simulink model "LaserLight_Demo2"  (R2017b)
settings: Solver=VariableStepAuto  StartTime=0.0  StopTime=1  RelTol=1e-3
values from neighbouring files (symbols this model uses):
  BackEMF0 = 0.09331    [System.m]
  BackEMF1 = 0.001545    [System.m]
  D = 10    [CONSTANTS.m]
  Elec0d = [.00105 2.25]    [System.m]
  Elec0n = [1]    [System.m]
  Elec1d = [1]    [0Controller.m]    (also in System.m = [.00105 2.25])
  Elec1n = [1]    [0Controller.m]    (also in System.m)
  Mech0d = [1]    [0Controller.m]    (also in System.m = [0.0000002059 0.0000009585])
  Mech0n = [1]    [0Controller.m]    (also in System.m)
  Mech1d = [1]    [0Controller.m]    (also in System.m = [0.0000025152 0.00001854])
  Mech1n = [1]    [0Controller.m]    (also in System.m)
  TConst0 = 0.001574542    [System.m]
  TConst1 = 0.0193    [System.m]
libraries: simulink x6
settings Model: Creator=Jimmy  LastModifiedBy=jmvsu
settings CodeAppCC: StateflowObjectComments=on

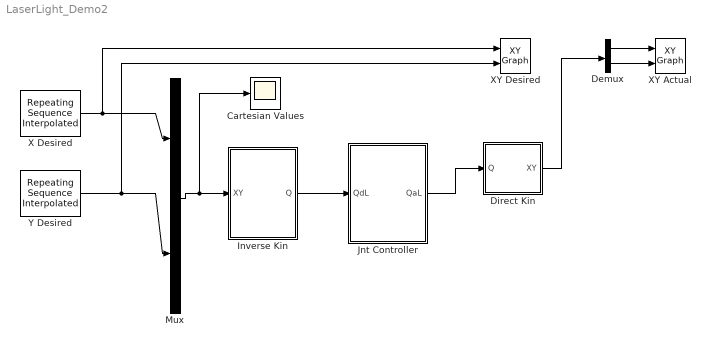
== system LaserLight_Demo2 ==
  Cartesian Values : Scope
  Demux : Demux  Outputs=2
  Direct Kin : Subsystem
  Inverse Kin : Subsystem
  Jnt Controller : Subsystem
  Mux : Mux  Inputs=2
  X Desired : simulink/Sources/Repeating Sequence Interpolated  OutValues=[100 100 -100 -100 100]  TimeValues=[0 0.25 0.5 0.75 1]  LookUpMeth=Interpolation-Use End Values  tsamp=0.01  OutMin=[]  OutMax=[]  OutDataTypeStr=double  OutputDataTypeScalingMode=double  OutDataType=fixdt(0,8)  OutScaling=2^-10
  XY Actual : simulink/Sinks/XY Graph  xmin=-125  xmax=125  ymin=-125  ymax=125  st=-1
  XY Desired : simulink/Sinks/XY Graph  xmin=-110  xmax=110  ymin=-110  ymax=110  st=-1
  Y Desired : simulink/Sources/Repeating Sequence Interpolated  OutValues=[-100 100 100 -100 -100]  TimeValues=[0 0.25 0.5 0.75 1]  LookUpMeth=Interpolation-Use End Values  tsamp=0.01  OutMin=[]  OutMax=[]  OutDataTypeStr=double  OutputDataTypeScalingMode=double  OutDataType=fixdt(0,8)  OutScaling=2^-10
  wires:
  Y Desired/1 -> XY Desired/2, Mux/2
  Demux/2 -> XY Actual/2
  Inverse Kin/1("Q ") -> Jnt Controller/1(QdL)
  Direct Kin/1(XY) -> Demux/1
  Jnt Controller/1(QaL) -> Direct Kin/1(Q)
  Demux/1 -> XY Actual/1
  Mux/1 -> Cartesian Values/1, Inverse Kin/1(XY)
  X Desired/1 -> Mux/1, XY Desired/1

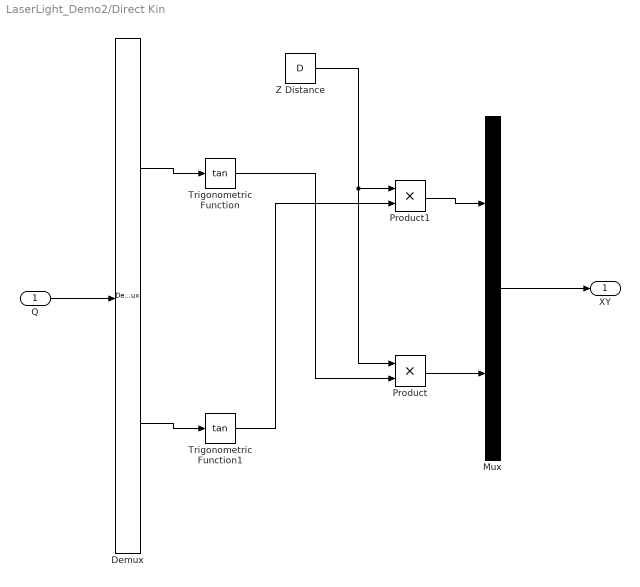
== system LaserLight_Demo2/Direct Kin ==
  Q : Inport
  Demux : Demux  Outputs=2
  Mux : Mux  Inputs=2
  Product : Product
  Product1 : Product
  Trigonometric Function : Trigonometry  Operator=tan
  Trigonometric Function1 : Trigonometry  Operator=tan
  Z Distance : Constant  Value=D
  XY : Outport
  wires:
  Q/1 -> Demux/1
  Mux/1 -> XY/1
  Demux/1 -> Trigonometric Function/1
  Demux/2 -> Trigonometric Function1/1
  Trigonometric Function/1 -> Product/2
  Z Distance/1 -> Product1/1, Product/1
  Trigonometric Function1/1 -> Product1/2
  Product1/1 -> Mux/1
  Product/1 -> Mux/2

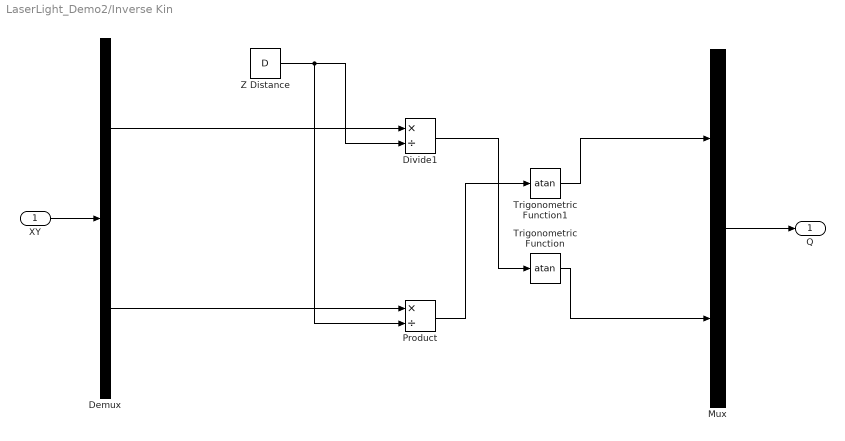
== system LaserLight_Demo2/Inverse Kin ==
  XY : Inport
  Demux : Demux  Outputs=2
  Divide1 : Product  Inputs=*/
  Mux : Mux  Inputs=2
  Product : Product  Inputs=*/
  Trigonometric Function : Trigonometry  Operator=atan
  Trigonometric Function1 : Trigonometry  Operator=atan
  "Z Distance " : Constant  Value=D
  "Q " : Outport
  wires:
  XY/1 -> Demux/1
  Mux/1 -> "Q "/1
  Demux/1 -> Divide1/1
  Trigonometric Function/1 -> Mux/2
  Divide1/1 -> Trigonometric Function/1
  "Z Distance "/1 -> Product/2, Divide1/2
  Demux/2 -> Product/1
  Trigonometric Function1/1 -> Mux/1
  Product/1 -> Trigonometric Function1/1

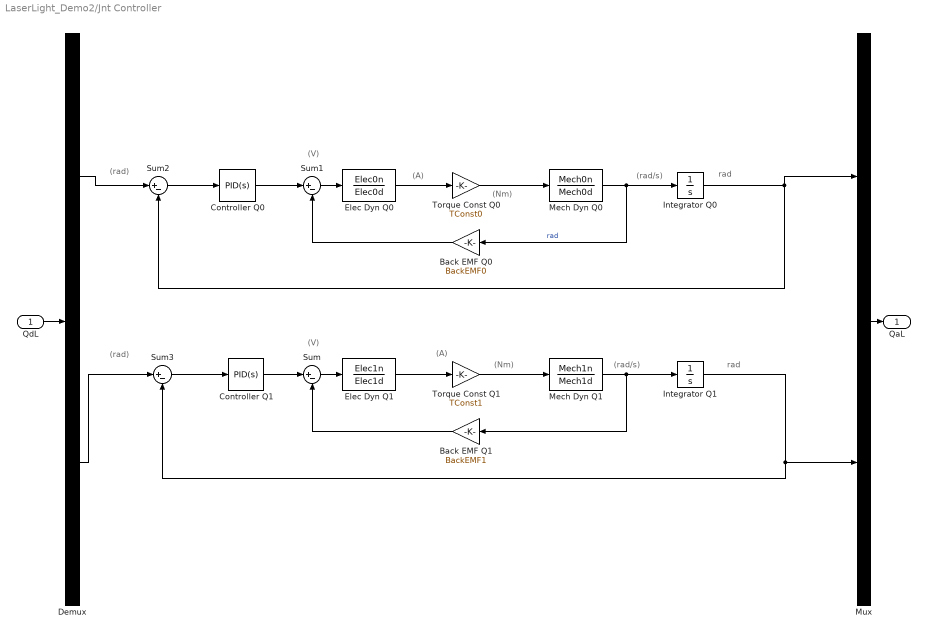
== system LaserLight_Demo2/Jnt Controller ==
  note: rad
  note: (rad/s)
  note: (V)
  note: (rad)
  note: (rad/s)
  note: (A)
  note: (Nm)
  note: (V)
  note: (A)
  note: (rad)
  note: (Nm)
  note: rad
  QdL : Inport
  Back EMF Q0 : Gain  Gain=BackEMF0
  Back EMF Q1 : Gain  Gain=BackEMF1
  Controller Q0 : simulink/Continuous/PID Controller  Controller=PID  TimeDomain=Continuous-time  SampleTime=-1  IntegratorMethod=Forward Euler  FilterMethod=Forward Euler  Form=Parallel  UseFilter=on  ControllerParametersSource=internal  P=1656.89310758008  I=104989.490543032  D=3.83138370012863  N=7457.36011167874  InitialConditionSource=internal  InitialConditionForIntegrator=0  InitialConditionForFilter=0  ExternalReset=none  LimitOutput=off  UpperSaturationLimit=inf  LowerSaturationLimit=-inf  LinearizeAsGain=on  AntiWindupMode=none  Kb=1  TrackingMode=off  Kt=1  PParamMin=[]  PParamMax=[]  IParamMin=[]  IParamMax=[]  DParamMin=[]  DParamMax=[]  NParamMin=[]  NParamMax=[]  KbParamMin=[]  KbParamMax=[]  KtParamMin=[]  KtParamMax=[]  POutMin=[]  POutMax=[]  IOutMin=[]  IOutMax=[]  DOutMin=[]  DOutMax=[]  NOutMin=[]  NOutMax=[]  KbOutMin=[]  KbOutMax=[]  KtOutMin=[]  KtOutMax=[]  IntegratorOutMin=[]  IntegratorOutMax=[]  FilterOutMin=[]  FilterOutMax=[]  SumOutMin=[]  SumOutMax=[]  SumI1OutMin=[]  SumI1OutMax=[]  SumI2OutMin=[]  SumI2OutMax=[]  SumI3OutMin=[]  SumI3OutMax=[]  SumDOutMin=[]  SumDOutMax=[]  SaturationOutMin=[]  SaturationOutMax=[]  IntegratorContinuousStateAttributes=''  IntegratorStateMustResolveToSignalObject=off  IntegratorRTWStateStorageClass=Auto  FilterContinuousStateAttributes=''  FilterStateMustResolveToSignalObject=off  FilterRTWStateStorageClass=Auto  DifferentiatorICPrevScaledInput=0  DifferentiatorOutMin=[]  DifferentiatorOutMax=[]  InitialConditionSetting=State (most efficient)  FilterDiffOutCoefMin=[]  FilterDiffOutCoefMax=[]  SumDenOutMin=[]  SumDenOutMax=[]  SumNumOutMin=[]  SumNumOutMax=[]  ReciprocalOutMin=[]  ReciprocalOutMax=[]  DivideOutMin=[]  DivideOutMax=[]  TunerSelectOption=Transfer Function Based (PID Tuner App)
  Controller Q1 : simulink/Continuous/PID Controller  Controller=PID  TimeDomain=Continuous-time  SampleTime=-1  IntegratorMethod=Forward Euler  FilterMethod=Forward Euler  Form=Parallel  UseFilter=on  ControllerParametersSource=internal  P=19.445961470142  I=200.878604706117  D=0.242603406733837  N=930.997703714061  InitialConditionSource=internal  InitialConditionForIntegrator=0  InitialConditionForFilter=0  ExternalReset=none  LimitOutput=off  UpperSaturationLimit=inf  LowerSaturationLimit=-inf  LinearizeAsGain=on  AntiWindupMode=none  Kb=1  TrackingMode=off  Kt=1  PParamMin=[]  PParamMax=[]  IParamMin=[]  IParamMax=[]  DParamMin=[]  DParamMax=[]  NParamMin=[]  NParamMax=[]  KbParamMin=[]  KbParamMax=[]  KtParamMin=[]  KtParamMax=[]  POutMin=[]  POutMax=[]  IOutMin=[]  IOutMax=[]  DOutMin=[]  DOutMax=[]  NOutMin=[]  NOutMax=[]  KbOutMin=[]  KbOutMax=[]  KtOutMin=[]  KtOutMax=[]  IntegratorOutMin=[]  IntegratorOutMax=[]  FilterOutMin=[]  FilterOutMax=[]  SumOutMin=[]  SumOutMax=[]  SumI1OutMin=[]  SumI1OutMax=[]  SumI2OutMin=[]  SumI2OutMax=[]  SumI3OutMin=[]  SumI3OutMax=[]  SumDOutMin=[]  SumDOutMax=[]  SaturationOutMin=[]  SaturationOutMax=[]  IntegratorContinuousStateAttributes=''  IntegratorStateMustResolveToSignalObject=off  IntegratorRTWStateStorageClass=Auto  FilterContinuousStateAttributes=''  FilterStateMustResolveToSignalObject=off  FilterRTWStateStorageClass=Auto  DifferentiatorICPrevScaledInput=0  DifferentiatorOutMin=[]  DifferentiatorOutMax=[]  InitialConditionSetting=State (most efficient)  FilterDiffOutCoefMin=[]  FilterDiffOutCoefMax=[]  SumDenOutMin=[]  SumDenOutMax=[]  SumNumOutMin=[]  SumNumOutMax=[]  ReciprocalOutMin=[]  ReciprocalOutMax=[]  DivideOutMin=[]  DivideOutMax=[]  TunerSelectOption=Transfer Function Based (PID Tuner App)
  Demux : Demux  Outputs=2
  Elec Dyn Q0 : TransferFcn  Numerator=Elec0n  Denominator=Elec0d
  Elec Dyn Q1 : TransferFcn  Numerator=Elec1n  Denominator=Elec1d
  Integrator Q0 : Integrator
  Integrator Q1 : Integrator
  Mech Dyn Q0 : TransferFcn  Numerator=Mech0n  Denominator=Mech0d
  Mech Dyn Q1 : TransferFcn  Numerator=Mech1n  Denominator=Mech1d
  Mux : Mux  Inputs=2
  Sum{,1..3} (4 alike) : Sum  Inputs=|+-
  Torque Const Q0 : Gain  Gain=TConst0
  Torque Const Q1 : Gain  Gain=TConst1
  QaL : Outport
  wires:
  QdL/1 -> Demux/1
  Mux/1 -> QaL/1
  Elec Dyn Q0/1 -> Torque Const Q0/1
  Mech Dyn Q1/1 -> Integrator Q1/1, Back EMF Q1/1
  Sum/1 -> Elec Dyn Q1/1
  Torque Const Q0/1 -> Mech Dyn Q0/1
  Mech Dyn Q0/1 -> Integrator Q0/1, Back EMF Q0/1  "rad"
  Sum3/1 -> Controller Q1/1
  Torque Const Q1/1 -> Mech Dyn Q1/1
  Sum1/1 -> Elec Dyn Q0/1
  Demux/2 -> Sum3/1
  Back EMF Q0/1 -> Sum1/2
  Integrator Q1/1 -> Sum3/2, Mux/2
  Back EMF Q1/1 -> Sum/2
  Controller Q0/1 -> Sum1/1
  Elec Dyn Q1/1 -> Torque Const Q1/1
  Demux/1 -> Sum2/1
  Integrator Q0/1 -> Sum2/2, Mux/1
  Controller Q1/1 -> Sum/1
  Sum2/1 -> Controller Q0/1
